simulink model "laneKeepingArcSplinesNestedRoad_2013a"  (R2013a)
settings: Solver=ode45  StartTime=0.0  StopTime=124  MaxStep=.1  RelTol=1e-3
values from neighbouring files (symbols this model uses):
  a = 1.421    [decouplingParametersNested.m]
  accGain = 1    [exampleRoad1.m]
  b = 1.029    [decouplingParametersNested.m]
  B = 8.22    [decouplingParametersNested.m]
  C = 1.65    [decouplingParametersNested.m]
  cf = -1.5e5*1    (= -150000)    [decouplingParametersNested.m]
  CircleData = [CircleData [CircleDataNew;pointCount:pointCount+size(CircleDataNew,2)-1] ]    [clothoidLCComputation.m]    (also in discreteClothoid.m = [CircleData [CX; CY; Rvec(j); phi(1); phi(end); S/2/n] ]; discreteClothoid_omer.m = [CircleData [CX; CY; Rvec(j); phi(1); phi(end); S/2/n] ]; exampleRoad1.m; exampleRoad2.m = [CircleData CircleDataNew])
  cr = -1.5e5*1    (= -150000)    [decouplingParametersNested.m]
  D = -muVal*m*g    [decouplingParametersNested.m]
  dpsi0 = 0    [decouplingParametersNested.m]
  dx0 = v    [decouplingParametersNested.m]
  dy0 = 0    [decouplingParametersNested.m]
  g = 9.81    [decouplingParametersNested.m]    (also in exampleRoad1.m; exampleroad_atakan.m; exampleroad_omer.m)
  Izz = 1950    [decouplingParametersNested.m]
  K = freqresp(G1,0)    [decouplingParametersNested.m]
  kappaf = 0    [decouplingParametersNested.m]
  Kd = 0.05    [decouplingParametersNested.m]
  KI1 = 10    [decouplingParametersNested.m]
  KI2 = 0.01    [decouplingParametersNested.m]
  KI3 = 0.01    [decouplingParametersNested.m]
  KP1 = 20    [decouplingParametersNested.m]
  KP2 = 30    [decouplingParametersNested.m]
  l_S = 1.25    [decouplingParametersNested.m]
  LineData = [LineData [LineDataNew; pointCount:pointCount+size(LineDataNew,2)-1] ]    [clothoidLCComputation.m]    (also in discreteClothoid.m = [LineData [CX; CY; AX(end); AY(end); S/2/n] ]; discreteClothoid_omer.m = [LineData [CX; CY; AX(end); AY(end); S/2/n] ]; exampleRoad1.m = [LineData [LineDataNew;pointCount:pointCount+size(LineDataNe; exampleRoad2.m = [LineData LineDataNew])
  m = 1480    [decouplingParametersNested.m]
  muVal = .82    (= 0.82)    [exampleRoad1.m]    (also in exampleroad_atakan.m; exampleroad_omer.m; parameterSelection.m = 0.5; parameterSelectionAnalytical.m)
  tau = 0.01    [decouplingParametersNested.m]
  v = v0    [decouplingParametersNested.m]
  y0 = 0    [decouplingParametersNested.m]
undefined symbols (not defined in the file or in its folder): Kd1, Kp1, Kp2, magnitude
settings Model: Creator=kws  LastModifiedBy=klaus
settings DataIOCC: SignalLoggingSaveFormat=ModelDataLogs
settings OptimizationCC: ExpressionDepthLimit=2147483647
settings DebuggingCC: MultiTaskDSMMsg=warning  MultiTaskCondExecSysMsg=none  FcnCallInpInsideContextMsg=EnableAllAsWarning  FrameProcessingCompatibilityMsg=error
settings GRTTargetCC: CodeReplacementLibrary=C89/C90 (ANSI)  CombineOutputUpdateFcns=off  GRTInterface=on

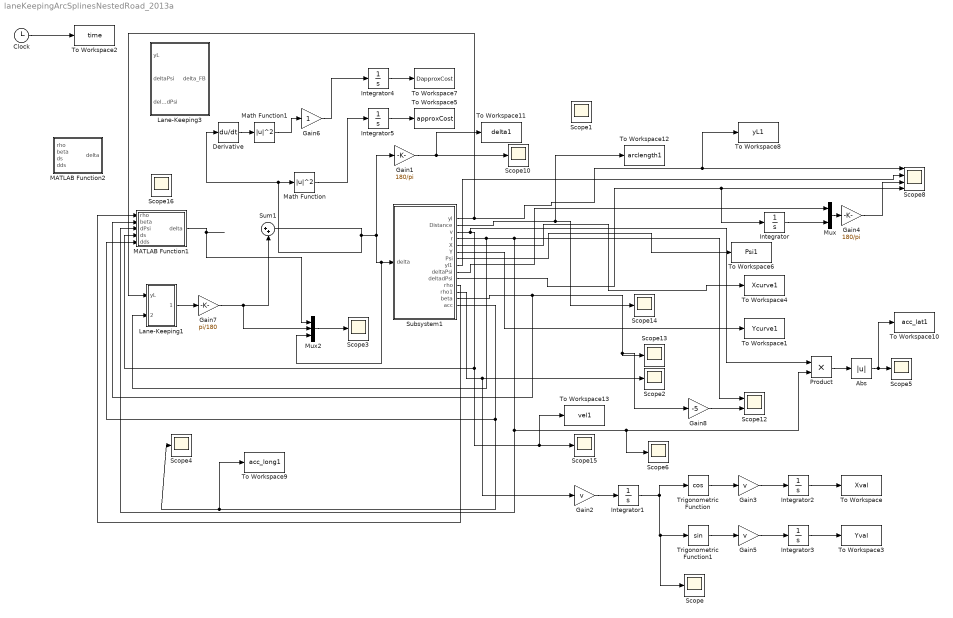
== system laneKeepingArcSplinesNestedRoad_2013a ==
  Abs : Abs
  Clock : Clock
  Derivative : Derivative
  Gain1 : Gain  Gain=180/pi
  Gain2 : Gain  Gain=v
  Gain3 : Gain  Gain=v
  Gain4 : Gain  Gain=180/pi
  Gain5 : Gain  Gain=v
  Gain6 : Gain
  Gain7 : Gain  Gain=pi/180
  Gain8 : Gain  Gain=-5
  Integrator{,1..5} (6 alike) : Integrator
  Lane-Keeping1 : Subsystem
  Lane-Keeping3 : Subsystem
  MATLAB Function1 : MATLAB Function  TreatAsAtomicUnit=on
  MATLAB Function2 : MATLAB Function  TreatAsAtomicUnit=on
  Math Function : Math  Operator=magnitude^2  SaturateOnIntegerOverflow=on
  Math Function1 : Math  Operator=magnitude^2  SaturateOnIntegerOverflow=on
  Mux : Mux  Inputs=2
  Mux2 : Mux  Inputs=3
  Product : Product
  Scope{,1..6,10,13..16} (12 alike) : Scope
      Scope settings: YMin=-10  YMax=10
      Scope1 settings: YMin=-7574108207.11842  YMax=841567578.57484  SaveName=ScopeData31
      Scope10 settings: YMin=-4  SaveName=ScopeData14
      Scope13 settings: YMin=-0.10177  YMax=0.10159  SaveName=ScopeData11
      Scope14 settings: YMin=1190.75  YMax=1194.5  SaveName=ScopeData8
      Scope15 settings: YMin=25  YMax=50
      Scope16 settings: TimeRange=24.1163  YMin=28.5  YMax=31.5  SaveName=ScopeData29
      Scope2 settings: YMin=-0.0125  YMax=0.0125  SaveName=ScopeData2
      Scope3 settings: YMin=-0.02  YMax=0.02  SaveName=ScopeData3
      Scope4 settings: YMin=-1  YMax=0.8  SaveName=ScopeData12
      Scope5 settings: YMin=0  YMax=3.75  SaveName=ScopeData17
      Scope6 settings: YMin=-0.08  YMax=0.09  SaveName=ScopeData18
  Scope12 : Scope  NumInputPorts=2
      settings: YMin=-0.54612~-5  YMax=0.54663~5  SaveName=ScopeData10
  Scope8 : Scope  NumInputPorts=4
      settings: YMin=-5.5~-5.5~-20000~-30  YMax=-4.6~-4.6~2500~-10  SaveName=ScopeData27
  Subsystem1 : Subsystem
  Sum1 : Sum  Inputs=|++
  To Workspace : ToWorkspace  VariableName=Xval  SampleTime=-1
  To Workspace1 : ToWorkspace  VariableName=Ycurve1  SampleTime=-1
  To Workspace10 : ToWorkspace  VariableName=acc_lat1  SampleTime=-1
  To Workspace11 : ToWorkspace  VariableName=delta1  SampleTime=-1
  To Workspace12 : ToWorkspace  VariableName=arclength1  SampleTime=-1
  To Workspace13 : ToWorkspace  VariableName=vel1  SampleTime=-1
  To Workspace2 : ToWorkspace  VariableName=time  SampleTime=-1
  To Workspace3 : ToWorkspace  VariableName=Yval  SampleTime=-1
  To Workspace4 : ToWorkspace  VariableName=Xcurve1  SampleTime=-1
  To Workspace5 : ToWorkspace  VariableName=approxCost  SampleTime=-1
  To Workspace6 : ToWorkspace  VariableName=Psi1  SampleTime=-1
  To Workspace7 : ToWorkspace  VariableName=DapproxCost  SampleTime=-1
  To Workspace8 : ToWorkspace  VariableName=yL1  SampleTime=-1
  To Workspace9 : ToWorkspace  VariableName=acc_long1  SampleTime=-1
  Trigonometric Function : Trigonometry  Operator=cos
  Trigonometric Function1 : Trigonometry
  wires:
  Clock/1 -> To Workspace2/1
  Subsystem1/7(Psi) -> To Workspace6/1
  Subsystem1/5(X) -> To Workspace4/1
  Gain1/1 -> To Workspace11/1, Scope10/1
  Subsystem1/8(yl1) -> Scope8/2
  Subsystem1/2(Distance) -> To Workspace12/1, Scope14/1
  Integrator/1 -> Mux/2
  Mux/1 -> Gain4/1
  Gain4/1 -> Scope8/3
  Subsystem1/10(deltadPsi) -> Scope8/4, Integrator/1
  Subsystem1/6(Y) -> To Workspace1/1
  Integrator1/1 -> Scope/1, Trigonometric Function1/1, Trigonometric Function/1
  Trigonometric Function/1 -> Gain3/1
  Trigonometric Function1/1 -> Gain5/1
  Integrator2/1 -> To Workspace/1
  Integrator3/1 -> To Workspace3/1
  Subsystem1/12(rho1) -> Gain2/1, Scope2/1
  Gain2/1 -> Integrator1/1
  Gain3/1 -> Integrator2/1
  Gain5/1 -> Integrator3/1
  Subsystem1/9(deltaPsi) -> Mux/1
  MATLAB Function1/1(delta) -> Mux2/1
  Subsystem1/4(r) -> Lane-Keeping1/2(dpsi), Scope6/1, Product/2, MATLAB Function1/3(dPsi), Scope12/1
  Subsystem1/13(beta) -> MATLAB Function1/2(beta), Gain8/1, Scope13/1
  Gain8/1 -> Scope12/2
  Mux2/1 -> Scope3/1
  Sum1/1 -> Math Function/1, Derivative/1, Mux2/3, Subsystem1/1(delta), Gain1/1
  Math Function/1 -> Integrator5/1
  Math Function1/1 -> Gain6/1
  Derivative/1 -> Math Function1/1
  Integrator5/1 -> To Workspace5/1
  Gain6/1 -> Integrator4/1
  Integrator4/1 -> To Workspace7/1
  Lane-Keeping1/1(delta_FB) -> Gain7/1
  Subsystem1/1(yl) -> Lane-Keeping1/1(yL), Scope8/1, To Workspace8/1
  Subsystem1/14(acc) -> MATLAB Function1/5(dds), To Workspace9/1, Scope4/1
  Subsystem1/3(v) -> Product/1, MATLAB Function1/4(ds), To Workspace13/1, Scope15/1
  Product/1 -> Abs/1
  Abs/1 -> To Workspace10/1, Scope5/1
  Subsystem1/11(rho) -> MATLAB Function1/1(rho)
  Gain7/1 -> Sum1/2, Mux2/2

== system laneKeepingArcSplinesNestedRoad_2013a/Lane-Keeping1 ==
  yL : Inport
  dpsi : Inport  Port=2
  C3 : Subsystem
  C4 : Subsystem
  Constant11 : Constant  Value=0
  Gain2 : Gain  Gain=K
  Scope7 : Scope
      settings: YMin=-0.35  YMax=0.35  SaveName=ScopeData5
  Sum2 : Sum  Inputs=+-|
  Sum3 : Sum  Inputs=|-+
  delta_FB : Outport
  wires:
  Sum2/1 -> C3/1(r)
  C4/1(delta_p) -> Gain2/1
  Gain2/1 -> Scope7/1, Sum2/2
  Constant11/1 -> Sum3/1
  C3/1(delta_f) -> delta_FB/1
  yL/1 -> Sum3/2
  Sum3/1 -> C4/1(e_y)
  dpsi/1 -> Sum2/1

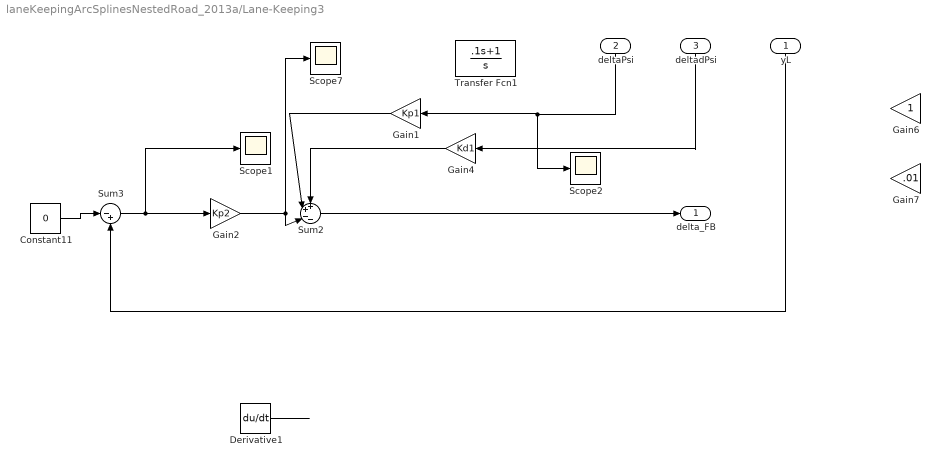
== system laneKeepingArcSplinesNestedRoad_2013a/Lane-Keeping3 ==
  yL : Inport
  deltaPsi : Inport  Port=2
  deltadPsi : Inport  Port=3
  Constant11 : Constant  Value=0
  Derivative1 : Derivative
  Gain1 : Gain  Gain=Kp1
  Gain2 : Gain  Gain=Kp2
  Gain4 : Gain  Gain=Kd1
  Gain6 : Gain
  Gain7 : Gain  Gain=.01
  Scope1 : Scope
      settings: YMin=11.2  YMax=11.625  SaveName=ScopeData37
  Scope2 : Scope
      settings: YMin=-0.04491  YMax=0.03856  SaveName=ScopeData30
  Scope7 : Scope
      settings: YMin=-0.10397  YMax=0.07071  SaveName=ScopeData5
  Sum2 : Sum  Inputs=++--
  Sum3 : Sum  Inputs=|-+
  Transfer Fcn1 : TransferFcn  Numerator=[.1 1]  Denominator=[1 0]
  delta_FB : Outport
  wires:
  deltaPsi/1 -> Scope2/1, Gain1/1
  Sum2/1 -> delta_FB/1
  Derivative1/1 -> ?
  Sum3/1 -> Scope1/1, Gain2/1
  Gain2/1 -> Sum2/3, Scope7/1
  deltadPsi/1 -> Gain4/1
  yL/1 -> Sum3/2
  Constant11/1 -> Sum3/1
  Gain1/1 -> Sum2/2
  Gain4/1 -> Sum2/1

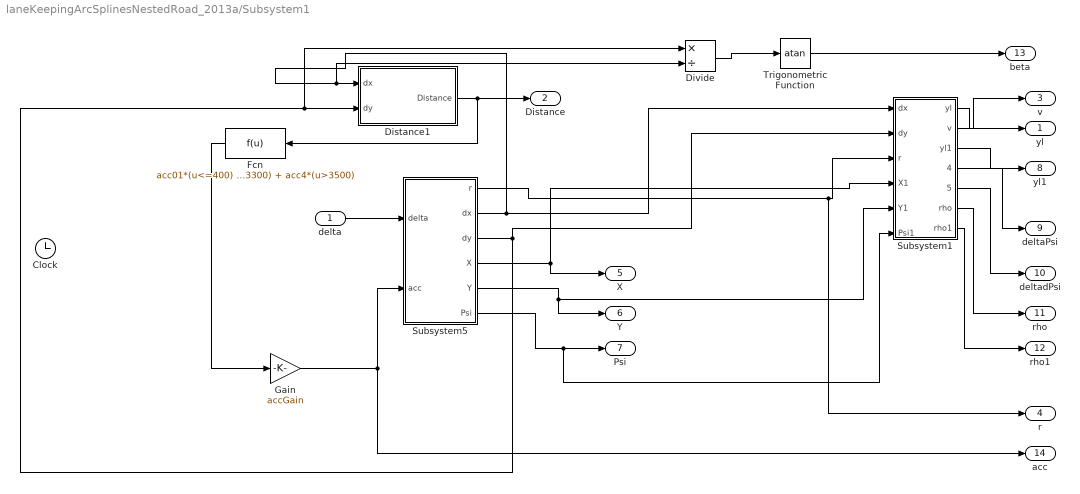
== system laneKeepingArcSplinesNestedRoad_2013a/Subsystem1 ==
  delta : Inport
  Clock : Clock
  Distance1 : Subsystem
  Divide : Product  Inputs=*/
  Fcn : Fcn  Expr=acc01*(u<=400) + acc1*(u>400&&u<=500) + acc12*(u>500&&u<=1050) + acc2*(u>1050&&u>=1250) + acc23*(u>1250&&u<=2000) + acc3*(u>2000&&u<=2150) + acc34*(u>2150&&u<=3300) + acc4*(u>3500)
  Gain : Gain  Gain=accGain
  Subsystem1 : Subsystem
  Subsystem5 : Subsystem
  Trigonometric Function : Trigonometry  Operator=atan
  yl : Outport
  Distance : Outport  Port=2
  v : Outport  Port=3
  r : Outport  Port=4
  X : Outport  Port=5
  Y : Outport  Port=6
  Psi : Outport  Port=7
  yl1 : Outport  Port=8
  deltaPsi : Outport  Port=9
  deltadPsi : Outport  Port=10
  rho : Outport  Port=11
  rho1 : Outport  Port=12
  beta : Outport  Port=13
  acc : Outport  Port=14
  wires:
  Subsystem1/1(yl) -> yl/1
  Subsystem5/3(dy) -> Subsystem1/2(dy), Divide/1, Distance1/2(dy)
  Subsystem5/2(dx) -> Divide/2, Distance1/1("dx "), Subsystem1/1(dx)
  Distance1/1(Distance) -> Fcn/1, Distance/1
  Subsystem1/2(v) -> v/1
  delta/1 -> Subsystem5/1(delta)
  Subsystem5/1(r) -> r/1, Subsystem1/3(r)
  Subsystem5/4(X) -> X/1, Subsystem1/4(X1)
  Subsystem5/5(Y) -> Y/1, Subsystem1/5(Y1)
  Subsystem5/6(Psi) -> Subsystem1/6(Psi1), Psi/1
  Fcn/1 -> Gain/1
  Subsystem1/3(yl1) -> yl1/1
  Subsystem1/4(deltaPsi) -> deltaPsi/1
  Subsystem1/5(deltadPsi) -> deltadPsi/1
  Subsystem1/6(rho) -> rho/1
  Subsystem1/7(rho1) -> rho1/1
  Divide/1 -> Trigonometric Function/1
  Trigonometric Function/1 -> beta/1
  Gain/1 -> Subsystem5/2(acc), acc/1

== system laneKeepingArcSplinesNestedRoad_2013a/Lane-Keeping1/C3 ==
  r : Inport
  Gain : Gain  Gain=KI1
  Gain1 : Gain  Gain=KP1
  Gain2 : Gain  Gain=-1
  Integrator : Integrator
  Sum : Sum  Inputs=|++
  delta_f : Outport
  wires:
  Gain/1 -> Sum/1
  Integrator/1 -> Gain/1
  r/1 -> Gain1/1, Integrator/1
  Sum/1 -> Gain2/1
  Gain1/1 -> Sum/2
  Gain2/1 -> delta_f/1

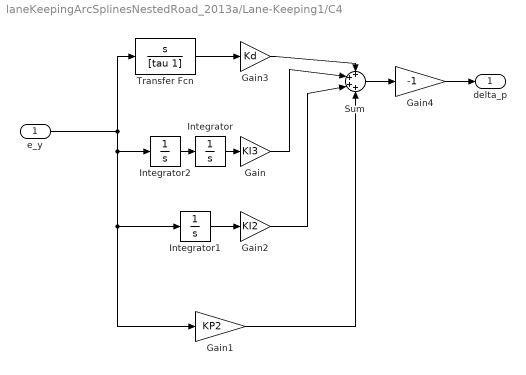
== system laneKeepingArcSplinesNestedRoad_2013a/Lane-Keeping1/C4 ==
  e_y : Inport
  Gain : Gain  Gain=KI3
  Gain1 : Gain  Gain=KP2
  Gain2 : Gain  Gain=KI2
  Gain3 : Gain  Gain=Kd
  Gain4 : Gain  Gain=-1
  Integrator : Integrator
  Integrator1 : Integrator
  Integrator2 : Integrator
  Sum : Sum  Inputs=++++
  Transfer Fcn : TransferFcn  Numerator=[1 0]  Denominator=[tau 1]
  delta_p : Outport
  wires:
  Sum/1 -> Gain4/1
  e_y/1 -> Transfer Fcn/1, Integrator1/1, Gain1/1, Integrator2/1
  Integrator/1 -> Gain/1
  Integrator1/1 -> Gain2/1
  Integrator2/1 -> Integrator/1
  Gain1/1 -> Sum/4
  Gain2/1 -> Sum/3
  Gain/1 -> Sum/2
  Transfer Fcn/1 -> Gain3/1
  Gain3/1 -> Sum/1
  Gain4/1 -> delta_p/1

== system laneKeepingArcSplinesNestedRoad_2013a/Subsystem1/Distance1 ==
  "dx " : Inport
  dy : Inport  Port=2
  Integrator : Integrator
  Math Function : Math  Operator=square  SaturateOnIntegerOverflow=on
  Math Function1 : Math  Operator=square  SaturateOnIntegerOverflow=on
  Sqrt : Sqrt  SaturateOnIntegerOverflow=on
  Sum : Sum  Inputs=|++
  Distance : Outport
  wires:
  "dx "/1 -> Math Function/1
  dy/1 -> Math Function1/1
  Math Function/1 -> Sum/1
  Math Function1/1 -> Sum/2
  Sum/1 -> Sqrt/1
  Sqrt/1 -> Integrator/1
  Integrator/1 -> Distance/1

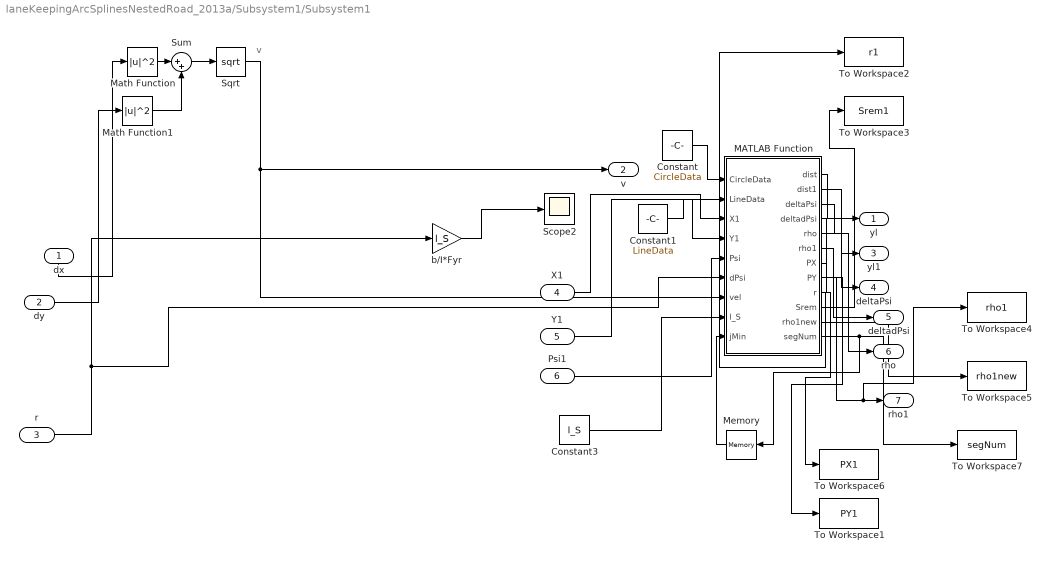
== system laneKeepingArcSplinesNestedRoad_2013a/Subsystem1/Subsystem1 ==
  note: v
  dx : Inport
  dy : Inport  Port=2
  r : Inport  Port=3
  X1 : Inport  Port=4
  Y1 : Inport  Port=5
  Psi1 : Inport  Port=6
  Constant : Constant  Value=CircleData
  Constant1 : Constant  Value=LineData
  Constant3 : Constant  Value=l_S
  MATLAB Function : MATLAB Function  TreatAsAtomicUnit=on
  Math Function : Math  Operator=magnitude^2  SaturateOnIntegerOverflow=on
  Math Function1 : Math  Operator=magnitude^2  SaturateOnIntegerOverflow=on
  Memory : Memory  X0=1
  Scope2 : Scope
      settings: TimeRange=30  YMin=-36000  YMax=-15000  SaveName=ScopeData28
  Sqrt : Sqrt  SaturateOnIntegerOverflow=on
  Sum : Sum  Inputs=|++
  To Workspace1 : ToWorkspace  VariableName=PY1  SampleTime=-1
  To Workspace2 : ToWorkspace  VariableName=r1  SampleTime=-1
  To Workspace3 : ToWorkspace  VariableName=Srem1  SampleTime=-1
  To Workspace4 : ToWorkspace  VariableName=rho1  SampleTime=-1
  To Workspace5 : ToWorkspace  VariableName=rho1new  SampleTime=-1
  To Workspace6 : ToWorkspace  VariableName=PX1  SampleTime=-1
  To Workspace7 : ToWorkspace  VariableName=segNum  SampleTime=-1
  b/I*Fyr : Gain  Gain=l_S
  yl : Outport
  v : Outport  Port=2
  yl1 : Outport  Port=3
  deltaPsi : Outport  Port=4
  deltadPsi : Outport  Port=5
  rho : Outport  Port=6
  rho1 : Outport  Port=7
  wires:
  dx/1 -> Math Function/1
  dy/1 -> Math Function1/1
  b/I*Fyr/1 -> Scope2/1
  Math Function1/1 -> Sum/2
  Sqrt/1 -> MATLAB Function/7(vel), v/1
  Math Function/1 -> Sum/1
  Sum/1 -> Sqrt/1
  r/1 -> MATLAB Function/6(dPsi), b/I*Fyr/1
  Constant/1 -> MATLAB Function/1(CircleData)
  Y1/1 -> MATLAB Function/4(Y1)
  Psi1/1 -> MATLAB Function/5(Psi)
  MATLAB Function/1(dist) -> yl/1
  X1/1 -> MATLAB Function/3(X1)
  Constant1/1 -> MATLAB Function/2(LineData)
  MATLAB Function/2(dist1) -> yl1/1
  MATLAB Function/3(deltaPsi) -> deltaPsi/1
  MATLAB Function/4(deltadPsi) -> deltadPsi/1
  Constant3/1 -> MATLAB Function/8(l_S)
  MATLAB Function/5(rho) -> rho/1
  MATLAB Function/6(rho1) -> To Workspace4/1, rho1/1
  MATLAB Function/7(PX) -> To Workspace6/1
  MATLAB Function/8(PY) -> To Workspace1/1
  MATLAB Function/10(Srem) -> To Workspace3/1
  MATLAB Function/9(r) -> To Workspace2/1
  MATLAB Function/11(rho1new) -> To Workspace5/1
  MATLAB Function/12(segNum) -> Memory/1, To Workspace7/1
  Memory/1 -> MATLAB Function/9(jMin)

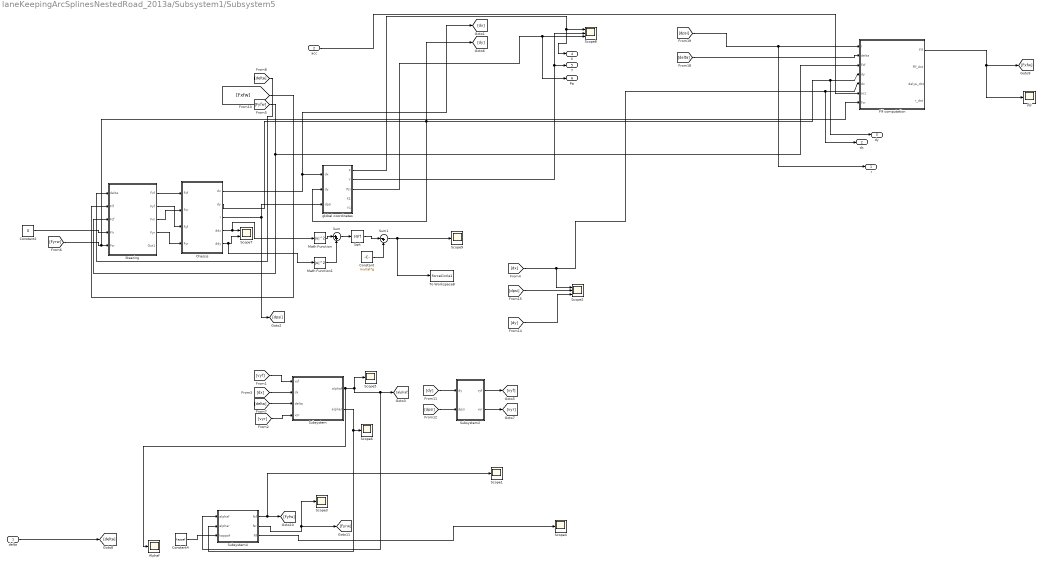
== system laneKeepingArcSplinesNestedRoad_2013a/Subsystem1/Subsystem5 ==
  delta : Inport
  acc : Inport  Port=2
  Alphaf : Scope
      settings: YMin=-10  YMax=10  SaveName=ScopeData13
  Chassis : Subsystem
  Constant : Constant  Value=muVal*g
  Constant2 : Constant  Value=0
  Constant4 : Constant  Value=kappaf
  Flf : Scope
      settings: YMin=-10  YMax=10  SaveName=ScopeData25
  Flf computation : Subsystem
  Math Function : Math  Operator=magnitude^2  SaturateOnIntegerOverflow=on
  Math Function1 : Math  Operator=magnitude^2  SaturateOnIntegerOverflow=on
  Scope{1,3..6,9} (6 alike) : Scope
      Scope1 settings: TimeRange=30  YMin=-12547.8136  YMax=12624.18485  SaveName=ScopeData3
      Scope3 settings: TimeRange=10  YMin=-13648.26805  YMax=13615.50136  SaveName=ScopeData4
      Scope4 settings: TimeRange=30  YMin=1336.33  YMax=1336.72  SaveName=ScopeData5
      Scope5 settings: TimeRange=30  YMin=-0.08416  YMax=0.08365  SaveName=ScopeData6
      Scope6 settings: TimeRange=30  YMin=-0.11424  YMax=0.11423  SaveName=ScopeData7
      Scope9 settings: TimeRange=9.24214  YMin=-13  SaveName=ScopeData16
  Scope2 : Scope  NumInputPorts=3
      settings: TimeRange=30  YMin=-1250~-1250~-900  YMax=1500~1250~700  SaveName=ScopeData2
  Scope7 : Scope  NumInputPorts=2
      settings: TimeRange=10  YMin=78.9932~28.5355  YMax=78.9938~28.5361  SaveName=ScopeData15
  Scope8 : Scope  NumInputPorts=3
      settings: TimeRange=10  YMin=78.9932~28.5355~0.835441  YMax=78.9938~28.5361~0.835451  SaveName=ScopeData10
  Sqrt : Sqrt  SaturateOnIntegerOverflow=on
  Steering : Subsystem
  Subsystem : Subsystem
  Subsystem2 : Subsystem
  Subsystem4 : Subsystem
  Sum : Sum  Inputs=|++
  Sum1 : Sum  Inputs=|-+
  To Workspace8 : ToWorkspace  VariableName=forceCircle1  SampleTime=-1
  global coordinates : Subsystem
  r : Outport
  dx : Outport  Port=2
  dy : Outport  Port=3
  X : Outport  Port=4
  Y : Outport  Port=5
  Psi : Outport  Port=6
  wires:
  [Fyrw] -> Steering/5(Fcr), Flf computation/7(Fcr)
  [dx] -> Scope2/1, Flf computation/5(dx), dx/1
  Flf computation/1(Flf) -> [Fxfw], Flf/1
  [dy] -> Scope2/3
  [dpsi] -> Scope2/2
  acc/1 -> Flf computation/6(acc)
  [dx] -> Subsystem/2(dx)
  [dy] -> Subsystem2/1(dy)
  global coordinates/3(Psi) -> Psi/1, Scope8/3
  global coordinates/2(Y) -> Scope8/2, Y/1
  Subsystem2/1(vyf) -> [vyf]
  global coordinates/1(X) -> X/1, Scope8/1
  [delta] -> Subsystem/3(delta)
  Chassis/3(r) -> global coordinates/3(dpsi), [dpsi]
  delta/1 -> [delta]
  [delta] -> Flf computation/2(delta)
  [dpsi] -> Flf computation/1(r), r/1
  [dpsi] -> Subsystem2/2(dpsi)
  [vyr] -> Subsystem/4(vyr)
  [vyf] -> Subsystem/1(vyf)
  [Fxfw] -> Steering/2(Flf)
  Subsystem2/2(vyr) -> [vyr]
  Constant4/1 -> Subsystem4/3(kappaf)
  Subsystem/1(alphaf) -> Subsystem4/1(alphaf), [alphaf], Scope5/1, Alphaf/1
  Chassis/1(dx) -> global coordinates/1(dx), [dx]
  Steering/3(Fxr) -> Chassis/2(Fxr)
  Subsystem4/3(flf) -> Scope4/1
  Subsystem/2(alphar) -> Subsystem4/2(alphar), Scope6/1
  Subsystem4/1(fsf) -> [Fyfw], Scope1/1
  Steering/4(Fyr) -> Chassis/4(Fyr)
  Steering/1(Fxf) -> Chassis/1(Fxf)
  Subsystem4/2(fsr) -> Scope3/1, [Fyrw]
  [Fyfw] -> Steering/3(Fcf), Flf computation/3(Fcf)
  [delta] -> Steering/1(delta)
  Steering/2(Fyf) -> Chassis/3(Fyf)
  Chassis/2(dy) -> [dy], Flf computation/4(dy), dy/1, global coordinates/2(dy)
  Constant2/1 -> Steering/4(Flr)
  Chassis/4(ddx) -> Math Function/1, Scope7/1
  Chassis/5("ddy ") -> Math Function1/1, Scope7/2
  Math Function/1 -> Sum/1
  Math Function1/1 -> Sum/2
  Sum/1 -> Sqrt/1
  Sqrt/1 -> Sum1/1
  Constant/1 -> Sum1/2
  Sum1/1 -> Scope9/1, To Workspace8/1

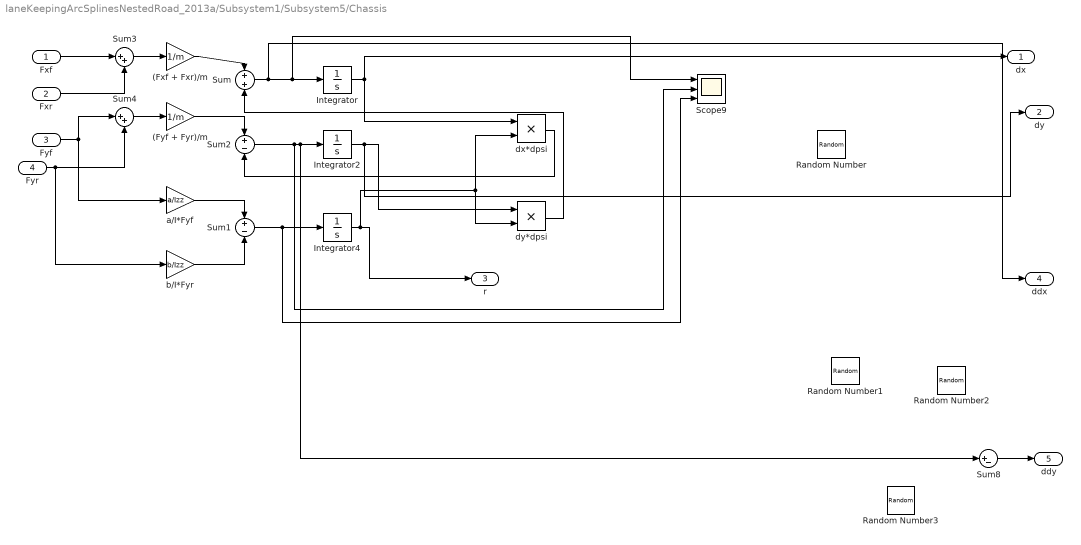
== system laneKeepingArcSplinesNestedRoad_2013a/Subsystem1/Subsystem5/Chassis ==
  Fxf : Inport
  Fxr : Inport  Port=2
  Fyf : Inport  Port=3
  Fyr : Inport  Port=4
  (Fxf + Fxr)/m : Gain  Gain=1/m
  (Fyf + Fyr)/m : Gain  Gain=1/m
  Integrator : Integrator  InitialCondition=dx0
  Integrator2 : Integrator  InitialCondition=dy0
  Integrator4 : Integrator  InitialCondition=dpsi0
  Random Number : RandomNumber  Variance=.001  Seed=1  SampleTime=.1
  Random Number1 : RandomNumber  Variance=.04  Seed=5
  Random Number2 : RandomNumber  Variance=.04  Seed=7
  Random Number3 : RandomNumber  Variance=.04  Seed=15
  Scope9 : Scope  NumInputPorts=3
      settings: TimeRange=30  YMin=-1250~-1250~-900  YMax=1500~1250~700  SaveName=ScopeData11
  Sum : Sum
  Sum1 : Sum  Inputs=+-
  Sum2 : Sum  Inputs=+-
  Sum3 : Sum  Inputs=|++
  Sum4 : Sum  Inputs=|++
  Sum8 : Sum  Inputs=|+-
  a/I*Fyf : Gain  Gain=a/Izz
  b/I*Fyr : Gain  Gain=b/Izz
  dx*dpsi : Product  RndMeth=Zero
  dy*dpsi : Product  RndMeth=Zero
  dx : Outport
  dy : Outport  Port=2
  r : Outport  Port=3
  ddx : Outport  Port=4
  "ddy " : Outport  Port=5
  wires:
  Integrator4/1 -> dx*dpsi/2, dy*dpsi/2, r/1
  Sum1/1 -> Integrator4/1, Scope9/3
  Sum2/1 -> Sum8/1, Integrator2/1, Scope9/2
  dx*dpsi/1 -> Sum2/2
  dy*dpsi/1 -> Sum/2
  (Fyf + Fyr)/m/1 -> Sum2/1
  (Fxf + Fxr)/m/1 -> Sum/1
  Sum3/1 -> (Fxf + Fxr)/m/1
  Sum4/1 -> (Fyf + Fyr)/m/1
  Fyf/1 -> Sum4/1, a/I*Fyf/1
  Fyr/1 -> Sum4/2, b/I*Fyr/1
  a/I*Fyf/1 -> Sum1/1
  b/I*Fyr/1 -> Sum1/2
  Fxf/1 -> Sum3/1
  Fxr/1 -> Sum3/2
  Integrator/1 -> dx/1, dx*dpsi/1
  Integrator2/1 -> dy/1, dy*dpsi/1
  Sum/1 -> ddx/1, Integrator/1, Scope9/1
  Sum8/1 -> "ddy "/1

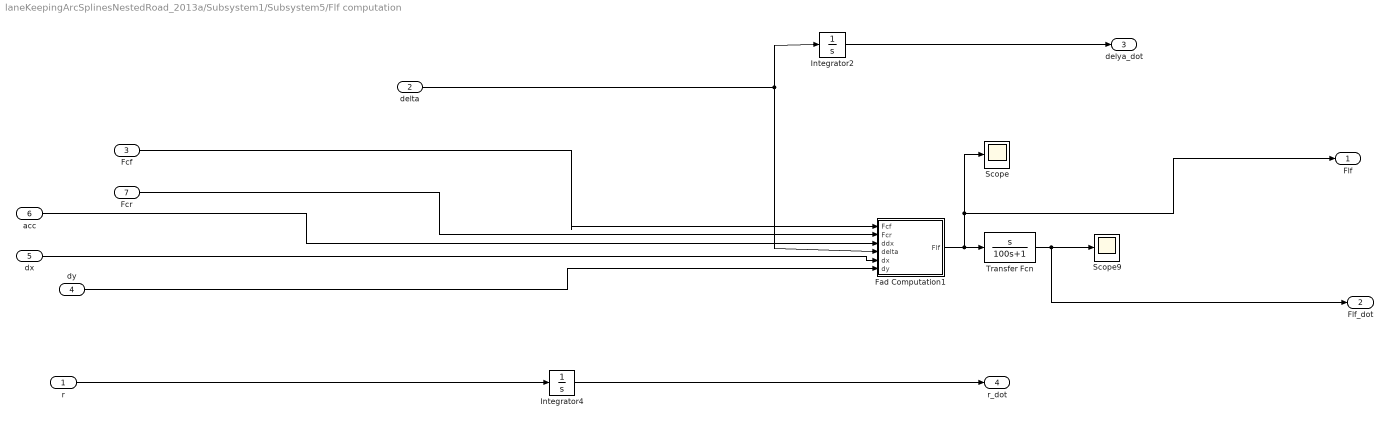
== system laneKeepingArcSplinesNestedRoad_2013a/Subsystem1/Subsystem5/Flf computation ==
  r : Inport
  delta : Inport  Port=2
  Fcf : Inport  Port=3
  dy : Inport  Port=4
  dx : Inport  Port=5
  acc : Inport  Port=6
  Fcr : Inport  Port=7
  Fad Computation1 : MATLAB Function  TreatAsAtomicUnit=on
  Integrator2 : Integrator
  Integrator4 : Integrator
  Scope : Scope
      settings: YMin=-11.23327  YMax=101.09943  SaveName=ScopeData19
  Scope9 : Scope
      settings: YMin=-10  YMax=10  SaveName=ScopeData20
  Transfer Fcn : TransferFcn  Numerator=[1 0]  Denominator=[100 1]
  Flf : Outport
  Flf_dot : Outport  Port=2
  delya_dot : Outport  Port=3
  r_dot : Outport  Port=4
  wires:
  Fcr/1 -> Fad Computation1/2(Fcr)
  dy/1 -> Fad Computation1/6(dy)
  Fcf/1 -> Fad Computation1/1(Fcf)
  delta/1 -> Integrator2/1, Fad Computation1/4(delta)
  dx/1 -> Fad Computation1/5(dx)
  acc/1 -> Fad Computation1/3(ddx)
  r/1 -> Integrator4/1
  Transfer Fcn/1 -> Scope9/1, Flf_dot/1
  Integrator2/1 -> delya_dot/1
  Fad Computation1/1(Flf) -> Scope/1, Flf/1, Transfer Fcn/1
  Integrator4/1 -> r_dot/1

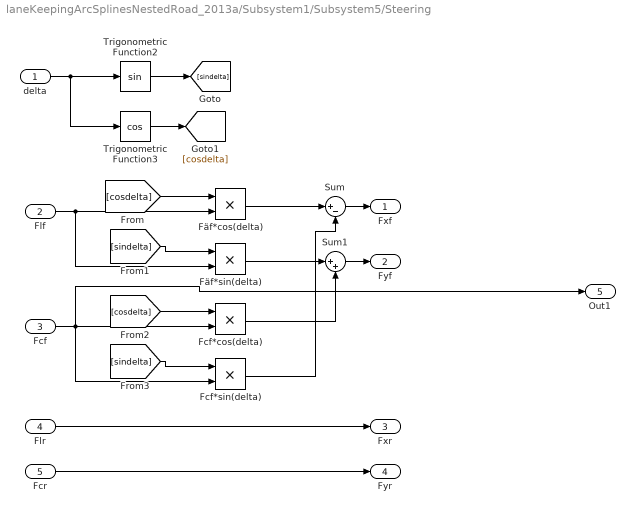
== system laneKeepingArcSplinesNestedRoad_2013a/Subsystem1/Subsystem5/Steering ==
  delta : Inport
  Flf : Inport  Port=2
  Fcf : Inport  Port=3
  Flr : Inport  Port=4
  Fcr : Inport  Port=5
  Fcf*cos(delta) : Product  RndMeth=Zero
  Fcf*sin(delta) : Product  RndMeth=Zero
  Fäf*cos(delta) : Product  RndMeth=Zero
  Fäf*sin(delta) : Product  RndMeth=Zero
  Sum : Sum  Inputs=|+-
  Sum1 : Sum  Inputs=|++
  Trigonometric Function2 : Trigonometry
  Trigonometric Function3 : Trigonometry  Operator=cos
  Fxf : Outport
  Fyf : Outport  Port=2
  Fxr : Outport  Port=3
  Fyr : Outport  Port=4
  Out1 : Outport  Port=5
  wires:
  Trigonometric Function2/1 -> [sindelta]
  Trigonometric Function3/1 -> [cosdelta]
  delta/1 -> Trigonometric Function2/1, Trigonometric Function3/1
  Flf/1 -> Fäf*cos(delta)/2, Fäf*sin(delta)/2
  [cosdelta] -> Fäf*cos(delta)/1
  [sindelta] -> Fäf*sin(delta)/1
  Fcf/1 -> Fcf*sin(delta)/2, Fcf*cos(delta)/2, Out1/1
  [cosdelta] -> Fcf*cos(delta)/1
  [sindelta] -> Fcf*sin(delta)/1
  Fäf*cos(delta)/1 -> Sum/1
  Fcf*sin(delta)/1 -> Sum/2
  Fäf*sin(delta)/1 -> Sum1/1
  Fcf*cos(delta)/1 -> Sum1/2
  Sum/1 -> Fxf/1
  Sum1/1 -> Fyf/1
  Flr/1 -> Fxr/1
  Fcr/1 -> Fyr/1

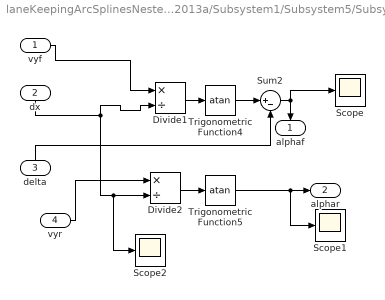
== system laneKeepingArcSplinesNestedRoad_2013a/Subsystem1/Subsystem5/Subsystem ==
  vyf : Inport
  dx : Inport  Port=2
  delta : Inport  Port=3
  vyr : Inport  Port=4
  Divide1 : Product  Inputs=*/
  Divide2 : Product  Inputs=*/
  Scope : Scope
      settings: TimeRange=30  YMin=0.00000008  YMax=0.00000037
  Scope1 : Scope
      settings: TimeRange=30  YMin=-1.5705  YMax=-1.57017
  Scope2 : Scope
      settings: TimeRange=30  YMin=0  YMax=1000  SaveName=ScopeData9
  Sum2 : Sum  Inputs=|+-
  Trigonometric Function4 : Trigonometry  Operator=atan
  Trigonometric Function5 : Trigonometry  Operator=atan
  alphaf : Outport
  alphar : Outport  Port=2
  wires:
  Trigonometric Function5/1 -> Scope1/1, alphar/1
  Trigonometric Function4/1 -> Sum2/1
  Divide1/1 -> Trigonometric Function4/1
  Sum2/1 -> Scope/1, alphaf/1
  Divide2/1 -> Trigonometric Function5/1
  dx/1 -> Divide1/2, Divide2/2, Scope2/1
  delta/1 -> Sum2/2
  vyf/1 -> Divide1/1
  vyr/1 -> Divide2/1

== system laneKeepingArcSplinesNestedRoad_2013a/Subsystem1/Subsystem5/Subsystem2 ==
  dy : Inport
  dpsi : Inport  Port=2
  Gain11 : Gain  Gain=a
  Gain12 : Gain  Gain=b
  Sum5 : Sum  Inputs=|++
  Sum6 : Sum  Inputs=|+-
  vyf : Outport
  vyr : Outport  Port=2
  wires:
  Gain11/1 -> Sum5/2
  Gain12/1 -> Sum6/2
  dy/1 -> Sum5/1, Sum6/1
  Sum5/1 -> vyf/1
  dpsi/1 -> Gain11/1, Gain12/1
  Sum6/1 -> vyr/1

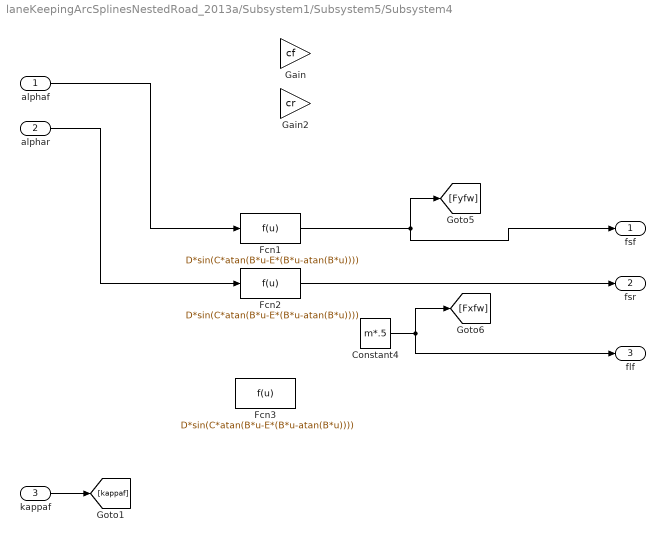
== system laneKeepingArcSplinesNestedRoad_2013a/Subsystem1/Subsystem5/Subsystem4 ==
  alphaf : Inport
  alphar : Inport  Port=2
  kappaf : Inport  Port=3
  Constant4 : Constant  Value=m*.5
  Fcn1 : Fcn  Expr=D*sin(C*atan(B*u-E*(B*u-atan(B*u))))
  Fcn2 : Fcn  Expr=D*sin(C*atan(B*u-E*(B*u-atan(B*u))))
  Fcn3 : Fcn  Expr=D*sin(C*atan(B*u-E*(B*u-atan(B*u))))
  Gain : Gain  Gain=cf
  Gain2 : Gain  Gain=cr
  fsf : Outport
  fsr : Outport  Port=2
  flf : Outport  Port=3
  wires:
  alphaf/1 -> Fcn1/1
  alphar/1 -> Fcn2/1
  kappaf/1 -> [kappaf]
  Constant4/1 -> flf/1, [Fxfw]
  Fcn1/1 -> [Fyfw], fsf/1
  Fcn2/1 -> fsr/1

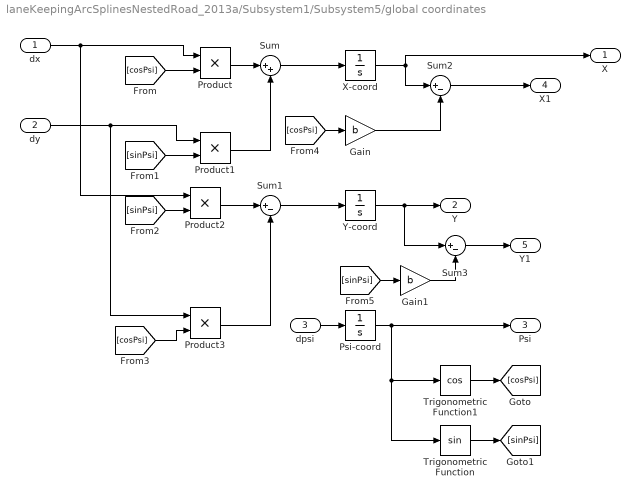
== system laneKeepingArcSplinesNestedRoad_2013a/Subsystem1/Subsystem5/global coordinates ==
  dx : Inport
  dy : Inport  Port=2
  dpsi : Inport  Port=3
  Gain : Gain  Gain=b
  Gain1 : Gain  Gain=b
  Product{,1..3} (4 alike) : Product  RndMeth=Zero
  Psi-coord : Integrator
  Sum : Sum  Inputs=|++
  Sum1 : Sum  Inputs=|+-
  Sum2 : Sum  Inputs=|+-
  Sum3 : Sum  Inputs=|+-
  Trigonometric Function : Trigonometry
  Trigonometric Function1 : Trigonometry  Operator=cos
  X-coord : Integrator
  Y-coord : Integrator  InitialCondition=y0
  X : Outport
  Y : Outport  Port=2
  Psi : Outport  Port=3
  X1 : Outport  Port=4
  Y1 : Outport  Port=5
  wires:
  [sinPsi] -> Gain1/1
  Gain1/1 -> Sum3/2
  Sum3/1 -> Y1/1
  Sum2/1 -> X1/1
  [cosPsi] -> Gain/1
  Gain/1 -> Sum2/2
  dpsi/1 -> Psi-coord/1
  Y-coord/1 -> Y/1, Sum3/1
  X-coord/1 -> Sum2/1, X/1
  [cosPsi] -> Product3/2
  [sinPsi] -> Product2/2
  [sinPsi] -> Product1/2
  [cosPsi] -> Product/2
  dy/1 -> Product3/1, Product1/1
  dx/1 -> Product2/1, Product/1
  Product3/1 -> Sum1/2
  Product1/1 -> Sum/2
  Product2/1 -> Sum1/1
  Product/1 -> Sum/1
  Sum1/1 -> Y-coord/1
  Sum/1 -> X-coord/1
  Trigonometric Function1/1 -> [cosPsi]
  Trigonometric Function/1 -> [sinPsi]
  Psi-coord/1 -> Trigonometric Function1/1, Trigonometric Function/1, Psi/1

== matlab function laneKeepingArcSplinesNestedRoad_2013a/MATLAB Function2 ==
  data: rho input; delta output; beta input; ds input; dds input
function delta = fcn(rho,beta,ds,dds)

aSym = 1.421;
bSym = 1.029;
mSym = 1480;
ISym = 1950;
cfSym = -1.5E5;
crSym = -1.5E5;
% dds = 0;
kSym = -4; %-2;
KSym = 2/5;

if rho == 0
    delta = 0;
elseif rho <= 0
    RSym = 1/rho;
    betaSym = beta;
%     delta = (1/rho*a*cf*atan(a*rho) - Izz*ddsVal + 1/rho*b*cr*atan(b*rho))/(1/rho*a*(cf - ddsVal*m));
%     delta = ((2*ISym^2*dds^2 + RSym^2*aSym^2*dds^2*mSym^2 + 2*RSym^2*bSym^2*crSym^2*atan(betaSym - bSym/RSym)^2 + RSym^2*aSym^2*cfSym^2*cos(betaSym)^2 + 4*ISym*RSym*bSym*crSym*dds*atan(betaSym - bSym/RSym) - 2*RSym^2*aSym^2*cfSym*dds*mSym*cos(betaSym) - 2*ISym*RSym*aSym*betaSym*dds^2*mSym + 2*ISym*RSym*aSym*betaSym*cfSym*dds*cos(betaSym) - 2*ISym*RSym*aSym*cfSym*dds*atan(betaSym + aSym/RSym)*cos(betaSym) - 2*RSym^2*aSym*bSym*betaSym*crSym*dds*mSym*atan(betaSym - bSym/RSym) + 2*RSym^2*aSym*bSym*betaSym*cfSym*crSym*atan(betaSym - bSym/RSym)*cos(betaSym) - 2*RSym^2*aSym*bSym*cfSym*crSym*atan(betaSym + aSym/RSym)*atan(betaSym - bSym/RSym)*cos(betaSym))^(1/2) + ISym*betaSym*dds + RSym*aSym*cfSym*cos(betaSym) - RSym*aSym*dds*mSym - RSym*bSym*betaSym*crSym*atan((bSym - RSym*betaSym)/RSym))/(ISym*dds - RSym*bSym*crSym*atan((bSym - RSym*betaSym)/RSym));
      delta = ((2*ISym^2*KSym^2*ds^2 + 2*ISym^2*RSym^2*betaSym^2*kSym^2 + RSym^2*aSym^2*dds^2*mSym^2 + 2*RSym^2*bSym^2*crSym^2*atan(betaSym - bSym/RSym)^2 + RSym^2*aSym^2*cfSym^2*cos(betaSym)^2 - 2*RSym^2*aSym^2*cfSym*dds*mSym*cos(betaSym) - 4*ISym^2*KSym*RSym*betaSym*ds*kSym + 4*ISym*KSym*RSym*bSym*crSym*ds*atan(betaSym - bSym/RSym) - 2*ISym*RSym^2*aSym*betaSym^2*cfSym*kSym*cos(betaSym) - 4*ISym*RSym^2*bSym*betaSym*crSym*kSym*atan(betaSym - bSym/RSym) + 2*ISym*RSym^2*aSym*betaSym^2*dds*kSym*mSym - 2*RSym^2*aSym*bSym*betaSym*crSym*dds*mSym*atan(betaSym - bSym/RSym) - 2*ISym*KSym*RSym*aSym*betaSym*dds*ds*mSym + 2*ISym*RSym^2*aSym*betaSym*cfSym*kSym*atan(betaSym + aSym/RSym)*cos(betaSym) + 2*RSym^2*aSym*bSym*betaSym*cfSym*crSym*atan(betaSym - bSym/RSym)*cos(betaSym) - 2*RSym^2*aSym*bSym*cfSym*crSym*atan(betaSym + aSym/RSym)*atan(betaSym - bSym/RSym)*cos(betaSym) + 2*ISym*KSym*RSym*aSym*betaSym*cfSym*ds*cos(betaSym) - 2*ISym*KSym*RSym*aSym*cfSym*ds*atan(betaSym + aSym/RSym)*cos(betaSym))^(1/2) + ISym*RSym*betaSym^2*kSym - RSym*aSym*cfSym*cos(betaSym) - ISym*KSym*betaSym*ds + RSym*aSym*dds*mSym + RSym*bSym*betaSym*crSym*atan((bSym - RSym*betaSym)/RSym))/(RSym*bSym*crSym*atan((bSym - RSym*betaSym)/RSym) - ISym*KSym*ds + ISym*RSym*betaSym*kSym);
else
    RSym = 1/rho;
    betaSym = beta;
%     delta =  -((2*ISym^2*dds^2 + RSym^2*aSym^2*dds^2*mSym^2 + 2*RSym^2*bSym^2*crSym^2*atan(betaSym - bSym/RSym)^2 + RSym^2*aSym^2*cfSym^2*cos(betaSym)^2 + 4*ISym*RSym*bSym*crSym*dds*atan(betaSym - bSym/RSym) - 2*RSym^2*aSym^2*cfSym*dds*mSym*cos(betaSym) - 2*ISym*RSym*aSym*betaSym*dds^2*mSym + 2*ISym*RSym*aSym*betaSym*cfSym*dds*cos(betaSym) - 2*ISym*RSym*aSym*cfSym*dds*atan(betaSym + aSym/RSym)*cos(betaSym) - 2*RSym^2*aSym*bSym*betaSym*crSym*dds*mSym*atan(betaSym - bSym/RSym) + 2*RSym^2*aSym*bSym*betaSym*cfSym*crSym*atan(betaSym - bSym/RSym)*cos(betaSym) - 2*RSym^2*aSym*bSym*cfSym*crSym*atan(betaSym + aSym/RSym)*atan(betaSym - bSym/RSym)*cos(betaSym))^(1/2) - ISym*betaSym*dds - RSym*aSym*cfSym*cos(betaSym) + RSym*aSym*dds*mSym + RSym*bSym*betaSym*crSym*atan((bSym - RSym*betaSym)/RSym))/(ISym*dds - RSym*bSym*crSym*atan((bSym - RSym*betaSym)/RSym));
    delta =  -((2*ISym^2*KSym^2*ds^2 + 2*ISym^2*RSym^2*betaSym^2*kSym^2 + RSym^2*aSym^2*dds^2*mSym^2 + 2*RSym^2*bSym^2*crSym^2*atan(betaSym - bSym/RSym)^2 + RSym^2*aSym^2*cfSym^2*cos(betaSym)^2 - 2*RSym^2*aSym^2*cfSym*dds*mSym*cos(betaSym) - 4*ISym^2*KSym*RSym*betaSym*ds*kSym + 4*ISym*KSym*RSym*bSym*crSym*ds*atan(betaSym - bSym/RSym) - 2*ISym*RSym^2*aSym*betaSym^2*cfSym*kSym*cos(betaSym) - 4*ISym*RSym^2*bSym*betaSym*crSym*kSym*atan(betaSym - bSym/RSym) + 2*ISym*RSym^2*aSym*betaSym^2*dds*kSym*mSym - 2*RSym^2*aSym*bSym*betaSym*crSym*dds*mSym*atan(betaSym - bSym/RSym) - 2*ISym*KSym*RSym*aSym*betaSym*dds*ds*mSym + 2*ISym*RSym^2*aSym*betaSym*cfSym*kSym*atan(betaSym + aSym/RSym)*cos(betaSym) + 2*RSym^2*aSym*bSym*betaSym*cfSym*crSym*atan(betaSym - bSym/RSym)*cos(betaSym) - 2*RSym^2*aSym*bSym*cfSym*crSym*atan(betaSym + aSym/RSym)*atan(betaSym - bSym/RSym)*cos(betaSym) + 2*ISym*KSym*RSym*aSym*betaSym*cfSym*ds*cos(betaSym) - 2*ISym*KSym*RSym*aSym*cfSym*ds*atan(betaSym + aSym/RSym)*cos(betaSym))^(1/2) - ISym*RSym*betaSym^2*kSym + RSym*aSym*cfSym*cos(betaSym) + ISym*KSym*betaSym*ds - RSym*aSym*dds*mSym - RSym*bSym*betaSym*crSym*atan((bSym - RSym*betaSym)/RSym))/(RSym*bSym*crSym*atan((bSym - RSym*betaSym)/RSym) - ISym*KSym*ds + ISym*RSym*betaSym*kSym);
end

== matlab function laneKeepingArcSplinesNestedRoad_2013a/Subsystem1/Subsystem1/MATLAB Function ==
  data: CircleData input; dist output; LineData input; X1 input; Y1 input; Psi input; dPsi input; vel input; l_S input; dist1 output; deltaPsi output; deltadPsi output; rho output; rho1 output; PX output; PY output; r output; Srem output; rho1new output; segNum output; jMin input
function [dist,dist1,deltaPsi,deltadPsi,rho,rho1,PX,PY,r,Srem,rho1new,segNum] = fcn(CircleData,LineData,X1,Y1,Psi,dPsi,vel,l_S,jMin)
%#codegen
a = 1.421;
b = 1.029;

dist = 1000000;
dist1 = 1000000;
deltaPsi = 0;
deltadPsi = 0;
CXvec = CircleData(1,:);
CYvec = CircleData(2,:);
Rvec = CircleData(3,:);
thetaSvec = CircleData(4,:);
thetaRvec = CircleData(5,:);
rho = 0;
rho1 = 0;
lineLength = 100;
Svec = LineData(1:2,:);
Evec = LineData(3:4,:);
segNum = 1;
psi1 = Psi;
Srem = l_S;

for j = 1:length(Rvec)
    % Compute angle of point P = (PX,PY)
    %     dir = -sign(Rvec(j))*[PX-CXvec(j);PY-CYvec(j)];
    theta1 = mod(atan2(sign(Rvec(j))*(X1-CXvec(j)),(-sign(Rvec(j))*(Y1-CYvec(j)))),2*pi);
    thetaRnew = mod(thetaRvec(j),2*pi);
    thetaSnew = mod(thetaSvec(j),2*pi);

    if thetaSvec(j) < thetaRvec(j)
        if thetaSnew < thetaRnew
            if theta1 < thetaSnew || theta1 >= thetaRnew
                continue;
            end
        else
           if theta1 < thetaSnew && theta1 > thetaRnew
               continue;
           end
        end
    else
        if thetaSnew > thetaRnew
            if theta1 > thetaSnew || theta1 <= thetaRnew
                continue;
            end
        else
           if theta1 > thetaSnew && theta1 < thetaRnew
               continue;
           end
        end    
    end
   % Compute normal vector
   distVec1 = [X1-CXvec(j); Y1-CYvec(j)];
   n1 = distVec1/sqrt(distVec1'*distVec1)*Rvec(j)/abs(Rvec(j));
   intVec1 = [CXvec(j);CYvec(j)]+Rvec(j)*n1;
   distNew1 = -([X1;Y1]-intVec1)'*n1;
   if abs(distNew1) < abs(dist1) % && CircleData(end,j) >= jMin
       rho1 = 1/Rvec(j);
       dist1 = distNew1;
       psi1 = theta1;
       segNum = CircleData(end,j);
        deltaPsi = (theta1-Psi);
        if thetaSvec(j) < thetaRvec(j) % increase in angle
            if theta1 > thetaRnew
                Srem = abs((thetaRnew+2*pi-theta1)*Rvec(j) );
            else
                Srem = abs((thetaRnew-theta1)*Rvec(j) );
            end
        else % decrease in angle
            if theta1 >  thetaRnew
                Srem = abs((thetaRnew-theta1)*Rvec(j) );
            else
                Srem = abs((thetaRnew-theta1-2*pi)*Rvec(j) );
            end
        end
%        deltadPsi = 1/Rvec(j)*vel-dPsi; % rho*v
%        if deltaPsi > pi
%            deltaPsi = deltaPsi-2*pi;
%        elseif deltaPsi < -pi
%            deltaPsi = deltaPsi+2*pi;
%        end
   end
%        plot([PX intVec(1)],[PY intVec(2)])

end

for j = 1:size(Svec,2)
    v = Evec(:,j)-Svec(:,j);
    n = [-v(2); v(1)]/norm(v);
    dir1 = [X1-Svec(1,j); Y1-Svec(2,j)];
    f = v'*dir1/norm(v)^2;
    if f < 0 || f > 1
        continue;
    else
        distNew1 = dir1'*n;
        if abs(distNew1) < abs(dist1) % && LineData(end,j) >= jMin
            rho1 = 0;
            dist1 = distNew1;
            segNum = LineData(end,j);
            Srem = (1-f)*LineData(5,j);
            psi1 = atan2(v(2),v(1));
             deltaPsi = (atan2(v(2),v(1))-Psi);
%             deltadPsi = -dPsi;
%             if deltaPsi > pi
%                 deltaPsi = deltaPsi-2*pi;
%             elseif deltaPsi < -pi
%                 deltaPsi = deltaPsi+2*pi;
%             end
        end
    end
end


lineIndex = find(LineData(end,:) == segNum+1);
if ~isempty(lineIndex)
   rho1new = 0;
else
   circleIndex = find(CircleData(end,:) == segNum+1);
   if isempty(circleIndex)
       rho1new = rho1;
   else
     rho1new = 1/CircleData(3,circleIndex(1));
   end
end

PX = X1+l_S*cos((psi1));
PY = Y1+l_S*sin((psi1)); 
alpha = 0;
r = 0;

if rho1 == 0 
    if Srem < l_S && rho1new ~= 0
        PX = X1+Srem*cos((psi1));
        PY = Y1+Srem*sin((psi1)); 
        r = 1/rho1new;
        alpha = (l_S-Srem)/r;
        PX = PX+r*(sin(psi1+alpha)-sin(psi1));
        PY = PY+r*(cos(psi1)-cos(psi1+alpha) );
    end
else
    if Srem >= l_S
        r = 1/rho1;
        alpha = l_S/r;
        PX = X1+r*(sin(psi1+alpha)-sin(psi1));     
        PY = Y1+r*(cos(psi1)-cos(psi1+alpha) );
    elseif rho1new == 0
        r = 1/rho1;
        alpha = Srem/r;
        PX = X1+r*(sin(psi1+alpha)-sin(psi1));
        PY = Y1+r*(cos(psi1)-cos(psi1+alpha) );
        PX = PX+(l_S-Srem)*cos((psi1+alpha));
        PY = PY+(l_S-Srem)*sin((psi1+alpha)); 
    else
        r = 1/rho1;
        alpha = Srem/r;
        PX = X1+r*(sin(psi1+alpha)-sin(psi1));
        PY = Y1+r*(cos(psi1)-cos(psi1+alpha) );
        r = 1/rho1new;
        psi1 = psi1+alpha;
        alpha = (l_S-Srem)/r;
        PX = PX+r*(sin(psi1+alpha)-sin(psi1));
        PY = PY+r*(cos(psi1)-cos(psi1+alpha) ); 
    end
end
    




for j = 1:length(Rvec)
    % Compute angle of point P = (PX,PY)
    %     dir = -sign(Rvec(j))*[PX-CXvec(j);PY-CYvec(j)];
    theta = mod(atan2(sign(Rvec(j))*(PX-CXvec(j)),(-sign(Rvec(j))*(PY-CYvec(j)))),2*pi);
    thetaRnew = mod(thetaRvec(j),2*pi);
    thetaSnew = mod(thetaSvec(j),2*pi);

    if thetaSvec(j) < thetaRvec(j)
        if thetaSnew < thetaRnew
            if theta < thetaSnew || theta >= thetaRnew
                continue;
            end
        else
           if theta < thetaSnew && theta > thetaRnew
               continue;
           end
        end
    else
        if thetaSnew > thetaRnew
            if theta > thetaSnew || theta <= thetaRnew
                continue;
            end
        else
           if theta > thetaSnew && theta < thetaRnew
               continue;
           end
        end    
    end
   % Compute normal vector
   distVec = [PX-CXvec(j); PY-CYvec(j)];
   n = distVec/sqrt(distVec'*distVec)*Rvec(j)/abs(Rvec(j));
   intVec = [CXvec(j);CYvec(j)]+Rvec(j)*n;
   distNew = -([PX;PY]-intVec)'*n;
   if abs(distNew) < abs(dist)
       rho = 1/Rvec(j);
       dist = distNew;
%        deltaPsi = (theta-Psi);
       deltadPsi = 1/Rvec(j)*vel-dPsi; % rho*v
       if deltaPsi > pi
           deltaPsi = deltaPsi-2*pi;
       elseif deltaPsi < -pi
           deltaPsi = deltaPsi+2*pi;
       end
   end
%        plot([PX intVec(1)],[PY intVec(2)])

end


for j = 1:size(Svec,2)
    v = Evec(:,j)-Svec(:,j);
    n = [-v(2); v(1)]/norm(v);
    dir = [PX-Svec(1,j); PY-Svec(2,j)];
    f = v'*dir/norm(v)^2;
    if f < 0 || f > 1
        continue;
    else
        distNew = dir'*n;
        if abs(distNew) < abs(dist)
            rho = 0;
            dist = distNew;
            lineLength = LineData(5,j);
%             deltaPsi = (atan2(v(2),v(1))-Psi);
            deltadPsi = -dPsi;
            if deltaPsi > pi
                deltaPsi = deltaPsi-2*pi;
            elseif deltaPsi < -pi
                deltaPsi = deltaPsi+2*pi;
            end
        end
    end
end
if rho1new == 0
    dist = 1*dist;
%     deltaPsi = .3*deltaPsi;
end
% if rho1 ~= 0
%     dist = 0;
%     deltaPsi = 0;
% end

== matlab function laneKeepingArcSplinesNestedRoad_2013a/MATLAB Function1 ==
  data: rho input; delta output; beta input; dPsi input; ds input; dds input
function delta = fcn(rho,beta,dPsi,ds,dds)

aSym = 1.421;
bSym = 1.029;
mSym = 1480;
ISym = 1950;
cfSym = -1.5E5;
crSym = -1.5E5;
% dds = 0;
kSym = .2; %-2;
KSym = .1;

if rho == 0
    delta = 0;
elseif rho > 0
    RSym = 1/rho;
    betaSym = beta;
    dPsiSym = dPsi;
%     delta = (1/rho*a*cf*atan(a*rho) - Izz*ddsVal + 1/rho*b*cr*atan(b*rho))/(1/rho*a*(cf - ddsVal*m));
%     delta = ((2*ISym^2*dds^2 + RSym^2*aSym^2*dds^2*mSym^2 + 2*RSym^2*bSym^2*crSym^2*atan(betaSym - bSym/RSym)^2 + RSym^2*aSym^2*cfSym^2*cos(betaSym)^2 + 4*ISym*RSym*bSym*crSym*dds*atan(betaSym - bSym/RSym) - 2*RSym^2*aSym^2*cfSym*dds*mSym*cos(betaSym) - 2*ISym*RSym*aSym*betaSym*dds^2*mSym + 2*ISym*RSym*aSym*betaSym*cfSym*dds*cos(betaSym) - 2*ISym*RSym*aSym*cfSym*dds*atan(betaSym + aSym/RSym)*cos(betaSym) - 2*RSym^2*aSym*bSym*betaSym*crSym*dds*mSym*atan(betaSym - bSym/RSym) + 2*RSym^2*aSym*bSym*betaSym*cfSym*crSym*atan(betaSym - bSym/RSym)*cos(betaSym) - 2*RSym^2*aSym*bSym*cfSym*crSym*atan(betaSym + aSym/RSym)*atan(betaSym - bSym/RSym)*cos(betaSym))^(1/2) + ISym*betaSym*dds + RSym*aSym*cfSym*cos(betaSym) - RSym*aSym*dds*mSym - RSym*bSym*betaSym*crSym*atan((bSym - RSym*betaSym)/RSym))/(ISym*dds - RSym*bSym*crSym*atan((bSym - RSym*betaSym)/RSym));
      delta = ((2*ISym^2*dds^2 + 2*ISym^2*ds^2*kSym^2 + 4*ISym^2*dds*ds*kSym + 2*ISym^2*RSym^2*dPsiSym^2*kSym^2 + RSym^2*aSym^2*dds^2*mSym^2 + 2*RSym^2*bSym^2*crSym^2*atan(betaSym - bSym/RSym)^2 + RSym^2*aSym^2*cfSym^2*cos(betaSym)^2 - 4*ISym^2*RSym*dPsiSym*dds*kSym - 4*ISym^2*RSym*dPsiSym*ds*kSym^2 + 4*ISym*RSym*bSym*crSym*dds*atan(betaSym - bSym/RSym) - 2*RSym^2*aSym^2*cfSym*dds*mSym*cos(betaSym) - 2*ISym*RSym*aSym*betaSym*dds^2*mSym + 4*ISym*RSym*bSym*crSym*ds*kSym*atan(betaSym - bSym/RSym) + 2*ISym*RSym*aSym*betaSym*cfSym*dds*cos(betaSym) - 2*ISym*RSym*aSym*cfSym*dds*atan(betaSym + aSym/RSym)*cos(betaSym) - 4*ISym*RSym^2*bSym*crSym*dPsiSym*kSym*atan(betaSym - bSym/RSym) - 2*RSym^2*aSym*bSym*betaSym*crSym*dds*mSym*atan(betaSym - bSym/RSym) - 2*ISym*RSym^2*aSym*betaSym*cfSym*dPsiSym*kSym*cos(betaSym) + 2*ISym*RSym^2*aSym*cfSym*dPsiSym*kSym*atan(betaSym + aSym/RSym)*cos(betaSym) + 2*RSym^2*aSym*bSym*betaSym*cfSym*crSym*atan(betaSym - bSym/RSym)*cos(betaSym) - 2*ISym*RSym*aSym*betaSym*dds*ds*kSym*mSym - 2*RSym^2*aSym*bSym*cfSym*crSym*atan(betaSym + aSym/RSym)*atan(betaSym - bSym/RSym)*cos(betaSym) + 2*ISym*RSym*aSym*betaSym*cfSym*ds*kSym*cos(betaSym) + 2*ISym*RSym^2*aSym*betaSym*dPsiSym*dds*kSym*mSym - 2*ISym*RSym*aSym*cfSym*ds*kSym*atan(betaSym + aSym/RSym)*cos(betaSym))^(1/2) + ISym*betaSym*dds + RSym*aSym*cfSym*cos(betaSym) + ISym*betaSym*ds*kSym - RSym*aSym*dds*mSym - RSym*bSym*betaSym*crSym*atan((bSym - RSym*betaSym)/RSym) - ISym*RSym*betaSym*dPsiSym*kSym)/(ISym*dds + ISym*ds*kSym - RSym*bSym*crSym*atan((bSym - RSym*betaSym)/RSym) - ISym*RSym*dPsiSym*kSym);
%     delta = ((2*ISym^2*dds^2 + 2*ISym^2*ds^2*kSym^2 + 4*ISym^2*dds*ds*kSym + 2*ISym^2*RSym^2*dPsiSym^2*kSym^2 + RSym^2*aSym^2*dds^2*mSym^2 + 2*RSym^2*bSym^2*crSym^2*atan((30*sin(betaSym) - bSym*dPsiSym)/(30*cos(betaSym)))^2 + RSym^2*aSym^2*cfSym^2*cos(betaSym)^2 - 4*ISym^2*RSym*dPsiSym*dds*kSym - 4*ISym^2*RSym*dPsiSym*ds*kSym^2 + 4*ISym*RSym*bSym*crSym*dds*atan((30*sin(betaSym) - bSym*dPsiSym)/(30*cos(betaSym))) - 2*RSym^2*aSym^2*cfSym*dds*mSym*cos(betaSym) - 2*ISym*RSym*aSym*betaSym*dds^2*mSym + 4*ISym*RSym*bSym*crSym*ds*kSym*atan((30*sin(betaSym) - bSym*dPsiSym)/(30*cos(betaSym))) + 2*ISym*RSym*aSym*betaSym*cfSym*dds*cos(betaSym) - 2*ISym*RSym*aSym*cfSym*dds*atan((30*sin(betaSym) + aSym*dPsiSym)/(30*cos(betaSym)))*cos(betaSym) - 4*ISym*RSym^2*bSym*crSym*dPsiSym*kSym*atan((30*sin(betaSym) - bSym*dPsiSym)/(30*cos(betaSym))) - 2*RSym^2*aSym*bSym*betaSym*crSym*dds*mSym*atan((30*sin(betaSym) - bSym*dPsiSym)/(30*cos(betaSym))) - 2*ISym*RSym^2*aSym*betaSym*cfSym*dPsiSym*kSym*cos(betaSym) + 2*ISym*RSym^2*aSym*cfSym*dPsiSym*kSym*atan((30*sin(betaSym) + aSym*dPsiSym)/(30*cos(betaSym)))*cos(betaSym) - 2*ISym*RSym*aSym*betaSym*dds*ds*kSym*mSym + 2*RSym^2*aSym*bSym*betaSym*cfSym*crSym*atan((30*sin(betaSym) - bSym*dPsiSym)/(30*cos(betaSym)))*cos(betaSym) - 2*RSym^2*aSym*bSym*cfSym*crSym*atan((30*sin(betaSym) + aSym*dPsiSym)/(30*cos(betaSym)))*atan((30*sin(betaSym) - bSym*dPsiSym)/(30*cos(betaSym)))*cos(betaSym) + 2*ISym*RSym*aSym*betaSym*cfSym*ds*kSym*cos(betaSym) + 2*ISym*RSym^2*aSym*betaSym*dPsiSym*dds*kSym*mSym - 2*ISym*RSym*aSym*cfSym*ds*kSym*atan((30*sin(betaSym) + aSym*dPsiSym)/(30*cos(betaSym)))*cos(betaSym))^(1/2) + ISym*betaSym*dds + RSym*aSym*cfSym*cos(betaSym) + ISym*betaSym*ds*kSym - RSym*aSym*dds*mSym - ISym*RSym*betaSym*dPsiSym*kSym + RSym*bSym*betaSym*crSym*atan((30*sin(betaSym) - bSym*dPsiSym)/(30*cos(betaSym))))/(ISym*dds + ISym*ds*kSym + RSym*bSym*crSym*atan((30*sin(betaSym) - bSym*dPsiSym)/(30*cos(betaSym))) - ISym*RSym*dPsiSym*kSym);
else
    RSym = 1/rho;
    betaSym = beta;
    dPsiSym = dPsi;
%     delta =  -((2*ISym^2*dds^2 + RSym^2*aSym^2*dds^2*mSym^2 + 2*RSym^2*bSym^2*crSym^2*atan(betaSym - bSym/RSym)^2 + RSym^2*aSym^2*cfSym^2*cos(betaSym)^2 + 4*ISym*RSym*bSym*crSym*dds*atan(betaSym - bSym/RSym) - 2*RSym^2*aSym^2*cfSym*dds*mSym*cos(betaSym) - 2*ISym*RSym*aSym*betaSym*dds^2*mSym + 2*ISym*RSym*aSym*betaSym*cfSym*dds*cos(betaSym) - 2*ISym*RSym*aSym*cfSym*dds*atan(betaSym + aSym/RSym)*cos(betaSym) - 2*RSym^2*aSym*bSym*betaSym*crSym*dds*mSym*atan(betaSym - bSym/RSym) + 2*RSym^2*aSym*bSym*betaSym*cfSym*crSym*atan(betaSym - bSym/RSym)*cos(betaSym) - 2*RSym^2*aSym*bSym*cfSym*crSym*atan(betaSym + aSym/RSym)*atan(betaSym - bSym/RSym)*cos(betaSym))^(1/2) - ISym*betaSym*dds - RSym*aSym*cfSym*cos(betaSym) + RSym*aSym*dds*mSym + RSym*bSym*betaSym*crSym*atan((bSym - RSym*betaSym)/RSym))/(ISym*dds - RSym*bSym*crSym*atan((bSym - RSym*betaSym)/RSym));
    delta =  -((2*ISym^2*dds^2 + 2*ISym^2*ds^2*kSym^2 + 4*ISym^2*dds*ds*kSym + 2*ISym^2*RSym^2*dPsiSym^2*kSym^2 + RSym^2*aSym^2*dds^2*mSym^2 + 2*RSym^2*bSym^2*crSym^2*atan(betaSym - bSym/RSym)^2 + RSym^2*aSym^2*cfSym^2*cos(betaSym)^2 - 4*ISym^2*RSym*dPsiSym*dds*kSym - 4*ISym^2*RSym*dPsiSym*ds*kSym^2 + 4*ISym*RSym*bSym*crSym*dds*atan(betaSym - bSym/RSym) - 2*RSym^2*aSym^2*cfSym*dds*mSym*cos(betaSym) - 2*ISym*RSym*aSym*betaSym*dds^2*mSym + 4*ISym*RSym*bSym*crSym*ds*kSym*atan(betaSym - bSym/RSym) + 2*ISym*RSym*aSym*betaSym*cfSym*dds*cos(betaSym) - 2*ISym*RSym*aSym*cfSym*dds*atan(betaSym + aSym/RSym)*cos(betaSym) - 4*ISym*RSym^2*bSym*crSym*dPsiSym*kSym*atan(betaSym - bSym/RSym) - 2*RSym^2*aSym*bSym*betaSym*crSym*dds*mSym*atan(betaSym - bSym/RSym) - 2*ISym*RSym^2*aSym*betaSym*cfSym*dPsiSym*kSym*cos(betaSym) + 2*ISym*RSym^2*aSym*cfSym*dPsiSym*kSym*atan(betaSym + aSym/RSym)*cos(betaSym) + 2*RSym^2*aSym*bSym*betaSym*cfSym*crSym*atan(betaSym - bSym/RSym)*cos(betaSym) - 2*ISym*RSym*aSym*betaSym*dds*ds*kSym*mSym - 2*RSym^2*aSym*bSym*cfSym*crSym*atan(betaSym + aSym/RSym)*atan(betaSym - bSym/RSym)*cos(betaSym) + 2*ISym*RSym*aSym*betaSym*cfSym*ds*kSym*cos(betaSym) + 2*ISym*RSym^2*aSym*betaSym*dPsiSym*dds*kSym*mSym - 2*ISym*RSym*aSym*cfSym*ds*kSym*atan(betaSym + aSym/RSym)*cos(betaSym))^(1/2) - ISym*betaSym*dds - RSym*aSym*cfSym*cos(betaSym) - ISym*betaSym*ds*kSym + RSym*aSym*dds*mSym + RSym*bSym*betaSym*crSym*atan((bSym - RSym*betaSym)/RSym) + ISym*RSym*betaSym*dPsiSym*kSym)/(ISym*dds + ISym*ds*kSym - RSym*bSym*crSym*atan((bSym - RSym*betaSym)/RSym) - ISym*RSym*dPsiSym*kSym);
%     delta = (ISym*betaSym*dds - (2*ISym^2*dds^2 + 2*ISym^2*ds^2*kSym^2 + 4*ISym^2*dds*ds*kSym + 2*ISym^2*RSym^2*dPsiSym^2*kSym^2 + RSym^2*aSym^2*dds^2*mSym^2 + 2*RSym^2*bSym^2*crSym^2*atan((30*sin(betaSym) - bSym*dPsiSym)/(30*cos(betaSym)))^2 + RSym^2*aSym^2*cfSym^2*cos(betaSym)^2 - 4*ISym^2*RSym*dPsiSym*dds*kSym - 4*ISym^2*RSym*dPsiSym*ds*kSym^2 + 4*ISym*RSym*bSym*crSym*dds*atan((30*sin(betaSym) - bSym*dPsiSym)/(30*cos(betaSym))) - 2*RSym^2*aSym^2*cfSym*dds*mSym*cos(betaSym) - 2*ISym*RSym*aSym*betaSym*dds^2*mSym + 4*ISym*RSym*bSym*crSym*ds*kSym*atan((30*sin(betaSym) - bSym*dPsiSym)/(30*cos(betaSym))) + 2*ISym*RSym*aSym*betaSym*cfSym*dds*cos(betaSym) - 2*ISym*RSym*aSym*cfSym*dds*atan((30*sin(betaSym) + aSym*dPsiSym)/(30*cos(betaSym)))*cos(betaSym) - 4*ISym*RSym^2*bSym*crSym*dPsiSym*kSym*atan((30*sin(betaSym) - bSym*dPsiSym)/(30*cos(betaSym))) - 2*RSym^2*aSym*bSym*betaSym*crSym*dds*mSym*atan((30*sin(betaSym) - bSym*dPsiSym)/(30*cos(betaSym))) - 2*ISym*RSym^2*aSym*betaSym*cfSym*dPsiSym*kSym*cos(betaSym) + 2*ISym*RSym^2*aSym*cfSym*dPsiSym*kSym*atan((30*sin(betaSym) + aSym*dPsiSym)/(30*cos(betaSym)))*cos(betaSym) - 2*ISym*RSym*aSym*betaSym*dds*ds*kSym*mSym + 2*RSym^2*aSym*bSym*betaSym*cfSym*crSym*atan((30*sin(betaSym) - bSym*dPsiSym)/(30*cos(betaSym)))*cos(betaSym) - 2*RSym^2*aSym*bSym*cfSym*crSym*atan((30*sin(betaSym) + aSym*dPsiSym)/(30*cos(betaSym)))*atan((30*sin(betaSym) - bSym*dPsiSym)/(30*cos(betaSym)))*cos(betaSym) + 2*ISym*RSym*aSym*betaSym*cfSym*ds*kSym*cos(betaSym) + 2*ISym*RSym^2*aSym*betaSym*dPsiSym*dds*kSym*mSym - 2*ISym*RSym*aSym*cfSym*ds*kSym*atan((30*sin(betaSym) + aSym*dPsiSym)/(30*cos(betaSym)))*cos(betaSym))^(1/2) + RSym*aSym*cfSym*cos(betaSym) + ISym*betaSym*ds*kSym - RSym*aSym*dds*mSym - ISym*RSym*betaSym*dPsiSym*kSym + RSym*bSym*betaSym*crSym*atan((30*sin(betaSym) - bSym*dPsiSym)/(30*cos(betaSym))))/(ISym*dds + ISym*ds*kSym + RSym*bSym*crSym*atan((30*sin(betaSym) - bSym*dPsiSym)/(30*cos(betaSym))) - ISym*RSym*dPsiSym*kSym);
end

== matlab function laneKeepingArcSplinesNestedRoad_2013a/Subsystem1/Subsystem5/Flf computation/Fad Computation1 ==
  data: Fcf input; Fcr input; ddx input; delta input; Flf output; dx input; dy input
function Flf = fcn(Fcf,Fcr,ddx,delta,dx,dy)
%#codegen
m = 1480;
 beta = atan(dy/dx);
 
 Flf = (m*ddx - Fcf*(cos(delta)*sin(beta) - sin(delta)*cos(beta))-Fcr*sin(beta))/(cos(delta)*cos(beta) + sin(delta)*sin(beta));
